simulink model "addr"  (Simulink 7.8)
settings: Solver=FixedStepDiscrete  StartTime=0.0  StopTime=10.0  RelTol=1e-3
libraries: rappid_ec_lib x13, rappid_lib x1, simulink x1
settings Model: Creator=Embed_Sys_course  LastModifiedBy=Embed_Sys_course
settings DataIOCC: ExternalInput=off  InitialState=off  SaveOutput=off  SignalLogging=off  SaveTime=off
settings OptimizationCC: InlineParams=on  OptimizeModelRefInitCode=on  LifeSpan=1
settings DebuggingCC: InheritedTsInSrcMsg=none  SingleTaskRateTransMsg=error  UnderSpecifiedDataTypeMsg=error  UnnecessaryDatatypeConvMsg=warning  UnconnectedInputMsg=error  UnconnectedOutputMsg=error  UnconnectedLineMsg=error  UnknownTsInhSupMsg=error
settings HardwareCC: ProdLargestAtomicInteger=Long  ProdLargestAtomicFloat=Double  ProdIntDivRoundTo=Zero  ProdEndianess=BigEndian  ProdHWDeviceType=Motorola PowerPC
settings RTWCC: SystemTargetFile=rappid.tlc  MakeCommand=rappid_make_rtw  TemplateMakefile=rappid_default_tmf  PostCodeGenCommand=rappid_analyzegencode(buildInfo)  Description=RAppID Toolbox MPC5554 Code Generation Target (rappid)  ProcessScript=rappid_make_rtw_hook
settings CodeAppCC: IgnoreCustomStorageClasses=off
settings STFCustomTargetCC: ModelReferenceCompliant=off  GeneratePreprocessorConditionals=Use local settings  CombineOutputUpdateFcns=on  ERTCustomFileBanners=on  SupportContinuousTime=off  SupportNonInlinedSFcns=off  SystemTargetFile=rappid.tlc
settings ERTTargetCC: MultiwordLength=2048  ModelReferenceCompliant=off  ParMdlRefBuildCompliant=off  CompOptLevelCompliant=off  ConcurrentExecutionCompliant=off  ERTFirstTimeCompliant=off  ModelStepFunctionPrototypeControlCompliant=off  CPPClassGenCompliant=off  InlinedParameterPlacement=NonHierarchical  ERTCustomFileTemplate=example_file_process.tlc  ConvertIfToSwitch=off  SuppressUnreachableDefaultCases=off

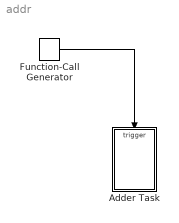
== system addr ==
  Adder Task : Subsystem
  Function-Call Generator : simulink/Ports & Subsystems/Function-Call Generator  sample_time=0.1  numberOfIterations=1
  wires:
  Function-Call Generator/1 -> Adder Task/Trigger

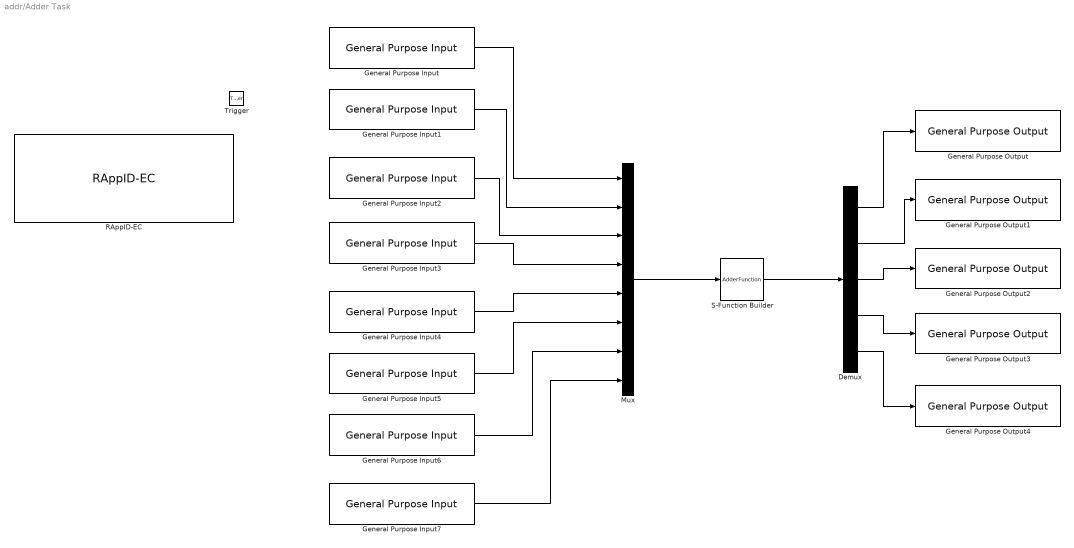
== system addr/Adder Task ==
  Trigger : TriggerPort  TriggerType=function-call  PortDimensions=1
  Demux : Demux  Outputs=5
  General Purpose Input : rappid_ec_lib/Peripheral Driver Blocks/GPIO Blocks/General Purpose Input  gpoi_inputs="93:   Primary Function \"DSPI SCKA\""  pinNum=93
  General Purpose Input1 : rappid_ec_lib/Peripheral Driver Blocks/GPIO Blocks/General Purpose Input  gpoi_inputs="94:   Primary Function \"DSPI SINA\""  pinNum=94
  General Purpose Input2 : rappid_ec_lib/Peripheral Driver Blocks/GPIO Blocks/General Purpose Input  gpoi_inputs="95:   Primary Function \"DSPI SOUTA\""  pinNum=95
  General Purpose Input3 : rappid_ec_lib/Peripheral Driver Blocks/GPIO Blocks/General Purpose Input  gpoi_inputs="96:   Primary Function \"DSPI PCSA0\""  pinNum=96
  General Purpose Input4 : rappid_ec_lib/Peripheral Driver Blocks/GPIO Blocks/General Purpose Input  gpoi_inputs="97:   Primary Function \"DSPI PCSA1\""  pinNum=97
  General Purpose Input5 : rappid_ec_lib/Peripheral Driver Blocks/GPIO Blocks/General Purpose Input  gpoi_inputs="98:   Primary Function \"DSPI PCSA2\""  pinNum=98
  General Purpose Input6 : rappid_ec_lib/Peripheral Driver Blocks/GPIO Blocks/General Purpose Input  gpoi_inputs="99:   Primary Function \"DSPI PCSA3\""  pinNum=99
  General Purpose Input7 : rappid_ec_lib/Peripheral Driver Blocks/GPIO Blocks/General Purpose Input  gpoi_inputs="100:   Primary Function \"DSPI PCSA4\""  pinNum=100
  General Purpose Output : rappid_ec_lib/Peripheral Driver Blocks/GPIO Blocks/General Purpose Output  gpoi_outputs="101:   Primary Function \"DSPI PCSA5\""  pinNum=101
  General Purpose Output1 : rappid_ec_lib/Peripheral Driver Blocks/GPIO Blocks/General Purpose Output  gpoi_outputs="102:   Primary Function \"DSPI SCKB\""  pinNum=102
  General Purpose Output2 : rappid_ec_lib/Peripheral Driver Blocks/GPIO Blocks/General Purpose Output  gpoi_outputs="103:   Primary Function \"DSPI SINB\""  pinNum=103
  General Purpose Output3 : rappid_ec_lib/Peripheral Driver Blocks/GPIO Blocks/General Purpose Output  gpoi_outputs="104:   Primary Function \"DSPI SOUTB\""  pinNum=104
  General Purpose Output4 : rappid_ec_lib/Peripheral Driver Blocks/GPIO Blocks/General Purpose Output  gpoi_outputs="105:   Primary Function \"DSPI PCSB0\""  pinNum=105
  Mux : Mux  Inputs=8
  RAppID-EC : rappid_lib/RAppID Initialization Blocks/RAppID-EC  Tag=RAppID  Priority=0  rtos=simpletarget  targetmcu=IntRAM  clockfrequency=128  basetaskpriority=20  systemcounter=0  systimer_isrpriority=1  systimer_period=0  isrstacksize=50  interruptdispatcher=None  stored_mdl_name=addr
  S-Function Builder : S-Function  InitFcn=try, set_param(gcb,'FunctionName','AdderFunction'), end  FunctionName=AdderFunction  SFunctionModules=AdderFunction_wrapper  WizardData=DataTag1  EnableBusSupport=off  mask(S-Function Builder){}
      mask help: Simulink:masks:SFunctionBuilder_MD
      mask init:
      | val = [[.9  0.75 0.75 1 1 .9 .9 1]',[1 1 0.75 0.75 .9 .9 1 .9]'];try , sys = get_param(gcb,'SfunBuilderFcnName');if isempty(sys), sys = get_param(gcb,'FunctionName'); end,catch, sys = get_param(gcb,'FunctionName'); end
      settings: CopyFcn=set_param(gcbh,'LinkStatus','none')  PreSaveFcn=try, set_param(gcb,'FunctionName','AdderFunction'), end  OpenFcn=sfunctionwizard(gcbh)
      mask Display: plot(val(:,1),val(:,2)),disp(sys), port_label('input',1,'u0'), port_label('output',1,'y0')
  wires:
  General Purpose Input/1 -> Mux/1
  General Purpose Input1/1 -> Mux/2
  General Purpose Input2/1 -> Mux/3
  General Purpose Input3/1 -> Mux/4
  General Purpose Input4/1 -> Mux/5
  General Purpose Input5/1 -> Mux/6
  General Purpose Input6/1 -> Mux/7
  General Purpose Input7/1 -> Mux/8
  Demux/1 -> General Purpose Output/1
  Demux/2 -> General Purpose Output1/1
  Demux/3 -> General Purpose Output2/1
  Demux/4 -> General Purpose Output3/1
  Demux/5 -> General Purpose Output4/1
  Mux/1 -> S-Function Builder/1
  S-Function Builder/1 -> Demux/1
